simulink model "IEEE123_4subsystem"  (R2022b)
settings: Solver=ode4  StartTime=0.0  StopTime=inf  FixedStep=Ts  MaxStep=1e-4  RelTol=1e-3
PreLoadFcn:
  | Ts = 50e-6;
PostLoadFcn:
  | Ts = 50e-6;
InitFcn:
  | %%%%%%%%%%%%%%%%%%%%%%%%
  | % Simulation data for the IEEE 123 Node Test Feeder model
  | %%%%%%%%%%%%%%%%%%%%%%%
  | 
  | % miles/km
  | mi2km = 1.60934;
  | 
  | % feet to km
  | ft2km = 0.0003048;
  | 
  | % microsiemens to Farads
  | ms2F = 1/2/pi/60*1e-6;
  | 
  | %% Configuration 1 - series reactance - ohm/mile
  | 
  | R_1 = [0.4576 0.1560 0.1535;0.1560 0.4666 0.1580;0.1535 0.1580 0.4615];
  | X_1 = [1.0780 0.5017 0.3849;0.5017 1.0482 0.4236;0.3849 0.4236 1.0651];
  | 
  | % charging susceptance - microsiemens/mile
  | 
  | B_1 = [5.6765 -1.8319 -0.6982;-1.8319 5.9809 -1.1645;-0.6982 -1.1645 5.3971];
  | 
  | % convert for SPS
  | 
  | R_1 = R_1/mi2km;
  | 
  | Rs_1=(R_1(1,1)+R_1(2,2)+R_1(3,3))/3;
  | Rm_1=(R_1(1,2)+R_1(1,3)+R_1(2,3))/3;
  | R1_1=Rs_1-Rm_1;
  | R0_1=Rs_1+2*Rm_1;
  | 
  | L_1 = X_1/mi2km/2/pi/60;
  | 
  | Ls_1=(L_1(1,1)+L_1(2,2)+L_1(3,3))/3;
  | Lm_1=(L_1(1,2)+L_1(1,3)+L_1(2,3))/3;
  | L1_1=Ls_1-Lm_1;
  | L0_1=Ls_1+2*Lm_1;
  | 
  | C_1 = B_1/mi2km*ms2F;
  | 
  | Cs_1=(C_1(1,1)+C_1(2,2)+C_1(3,3))/3;
  | Cm_1=(C_1(1,2)+C_1(1,3)+C_1(2,3))/3;
  | C1_1=Cs_1-Cm_1;
  | C0_1=Cs_1+2*Cm_1;
  | 
  | 
  | %% Configuration 2 - series reactance - ohm/mile
  | 
  | R_2 = [0.4666 0.1580 0.1560;0.1580 0.4615 0.1535;0.1560 0.1535 0.4576];
  | X_2 = [1.0482 0.4236 0.5017;0.4236 1.0651 0.3849;0.5017 0.3849 1.0780];
  | 
  | % charging susceptance - microsiemens/mile
  | 
  | B_2 = [5.9809 -1.1645 -1.8319;-1.1645 5.3971 -0.6982;-1.8319 -0.6982 5.6765];
  | 
  | % convert for SPS
  | 
  | R_2 = R_2/mi2km;
  | 
  | Rs_2=(R_2(1,1)+R_2(2,2)+R_2(3,3))/3;
  | ... (+341 lines)
undefined symbols (not defined in the file): D1, Delta, find_system, I, Left, MOV_segment9, powergui, Right, type, V, X
libraries: spsGroundLib x242, spsThreePhaseVIMeasurementLib x134, spsSeriesRLCBranchLib x107, spsSeriesRLCLoadLib x83, spsPiSectionLineLib x61, spsThreePhasePISectionLineLib x60, spsVoltageMeasurementLib x52, spsDCVoltageSourceLib x36, ssn_lib x28, artemis x24, spsACCurrentSourceLib x18, spsOnDelayLib x18
(part 7 of 15)

== system IEEE123_4subsystem/SS_123p2/Regulator3 ==
  Mux : Mux  Inputs=2
  Single Phase SVR_A : Subsystem  LoadFcn=find_system(gcs,'FollowLinks', 'on', 'LookUnderMasks', 'all');  mask(Single-Phase OLTC){pNom=5e6/3, fNom=60, vNom=4160/sqrt(3), ctRatio=50, ptRatio=20, DeltaU=0.00625, TapMinMax=[-16 16], InitialTap=0, TapSelectionTime=0.2, RegulatorOn=on, Regulator=[120/120  1/120  0.2], Comp=[0.4 0.4]}
      mask prompts: pNom "Nominal Power (VA)"; fNom "Nominal Frequency (Hz)"; vNom "Nominal Voltage (Vrms)"; ctRatio "Primary CT Rating (A)"; ptRatio "PT Ratio"; DeltaU "Voltage Step Per Tap (pu)"; TapMinMax "Minimum and Maximum Tap Positions"; InitialTap "Initial Tap Position"; TapSelectionTime "Tap Selection Time (s)"; RegulatorOn "Voltage Regulator"; Regulator "Voltage Regulator [ Vref(pu) DeadBand(pu)  Delay(s)]"; Comp "Compensator Settings [R (V) X(V)]"
      mask help:
      | Models a single-phase On Load Tap Changer (OLTC). The single-phase secondary of multi-tap winding is modeled with a Variable-Ratio Transformer block.
      |
      | The transformer voltage ratio U2/U1 (in pu) is given by:
      |                 U2/U1= 1+TapPosition*DeltaU
      | Tap position 0 corresponds to nominal voltage ratio.
      |
      | When Voltage regulator is 'on',  voltage regulator asks for a tap change if:
      |                  abs(Vm-Vref)>DeadBand/2  during a time  t > Delay.
      |
      | where 'Vm' is voltage measured at regulating point and Vref is reference voltage.
      | With line drop compensation, Vm=Vsec-Isec(R+jX)
      mask init:
      | RegulatorVref=Regulator(1);
      | RegulatorDeadBand=Regulator(2);
      | RegulatorDelay=Regulator(3);
      | Rc=Comp(1);
      | Xc=Comp(2);
      mask TypeOptions RegulatorOn: off | on
      mask Callback RegulatorOn:
      | tempMaskVis=get_param(gcb,'MaskVisibilities');
      | if strcmp(get_param(gcb,'RegulatorOn'),'on')
      | 	tempMaskVis{11}='on';
      | 	set_param(gcb,'MaskVisibilities',tempMaskVis);
      | else
      | 	tempMaskVis{11}='off';
      | 	set_param(gcb,'MaskVisibilities',tempMaskVis);
      | end
      | if strcmp(get_param(gcb,'RegulatorOn'),'on')
      | 	tempMaskVis{12}='on';
      | 	set_param(gcb,'MaskVisibilities',tempMaskVis);
      | else
      | 	tempMaskVis{12}='off';
      | 	set_param(gcb,'MaskVisibilities',tempMaskVis);
      | end
      mask DialogControl Container8 Prompt: Setup
      mask DialogControl Container13 Prompt: Regulator Parameters
      mask Display:
      | color('green');
      | r=50;x=40;y=80;
      | th = 0:pi/100:2*pi;
      | f = r * exp(j*th) + x+j*y;
      | plot(real(f), imag(f));
      | color('blue');
      | plot([-10 90],[30,130])
      | plot([75 90],[125,130])
      | plot([85 90],[115,130])
      | color('black')
      | port_label('Lconn',1,'S');port_label('Rconn',1,'L');
      | text(58,115,'Tap');
      | text(43,70,'Vsec');
      | text(48,95,'Isec');
  Single Phase SVR_C : Subsystem  LoadFcn=find_system(gcs,'FollowLinks', 'on', 'LookUnderMasks', 'all');  mask(Single-Phase OLTC){pNom=5e6/3, fNom=60, vNom=4160/sqrt(3), ctRatio=50, ptRatio=20, DeltaU=0.00625, TapMinMax=[-16 16], InitialTap=-1, TapSelectionTime=0.2, RegulatorOn=on, Regulator=[120/120  1/120  0.2], Comp=[0.4 0.4]}
      mask prompts: pNom "Nominal Power (VA)"; fNom "Nominal Frequency (Hz)"; vNom "Nominal Voltage (Vrms)"; ctRatio "Primary CT Rating (A)"; ptRatio "PT Ratio"; DeltaU "Voltage Step Per Tap (pu)"; TapMinMax "Minimum and Maximum Tap Positions"; InitialTap "Initial Tap Position"; TapSelectionTime "Tap Selection Time (s)"; RegulatorOn "Voltage Regulator"; Regulator "Voltage Regulator [ Vref(pu) DeadBand(pu)  Delay(s)]"; Comp "Compensator Settings [R (V) X(V)]"
      mask help:
      | Models a single-phase On Load Tap Changer (OLTC). The single-phase secondary of multi-tap winding is modeled with a Variable-Ratio Transformer block.
      |
      | The transformer voltage ratio U2/U1 (in pu) is given by:
      |                 U2/U1= 1+TapPosition*DeltaU
      | Tap position 0 corresponds to nominal voltage ratio.
      |
      | When Voltage regulator is 'on',  voltage regulator asks for a tap change if:
      |                  abs(Vm-Vref)>DeadBand/2  during a time  t > Delay.
      |
      | where 'Vm' is voltage measured at regulating point and Vref is reference voltage.
      | With line drop compensation, Vm=Vsec-Isec(R+jX)
      mask init:
      | RegulatorVref=Regulator(1);
      | RegulatorDeadBand=Regulator(2);
      | RegulatorDelay=Regulator(3);
      | Rc=Comp(1);
      | Xc=Comp(2);
      mask TypeOptions RegulatorOn: off | on
      mask Callback RegulatorOn:
      | tempMaskVis=get_param(gcb,'MaskVisibilities');
      | if strcmp(get_param(gcb,'RegulatorOn'),'on')
      | 	tempMaskVis{11}='on';
      | 	set_param(gcb,'MaskVisibilities',tempMaskVis);
      | else
      | 	tempMaskVis{11}='off';
      | 	set_param(gcb,'MaskVisibilities',tempMaskVis);
      | end
      | if strcmp(get_param(gcb,'RegulatorOn'),'on')
      | 	tempMaskVis{12}='on';
      | 	set_param(gcb,'MaskVisibilities',tempMaskVis);
      | else
      | 	tempMaskVis{12}='off';
      | 	set_param(gcb,'MaskVisibilities',tempMaskVis);
      | end
      mask DialogControl Container8 Prompt: Setup
      mask DialogControl Container13 Prompt: Regulator Parameters
      mask Display:
      | color('green');
      | r=50;x=40;y=80;
      | th = 0:pi/100:2*pi;
      | f = r * exp(j*th) + x+j*y;
      | plot(real(f), imag(f));
      | color('blue');
      | plot([-10 90],[30,130])
      | plot([75 90],[125,130])
      | plot([85 90],[115,130])
      | color('black')
      | port_label('Lconn',1,'S');port_label('Rconn',1,'L');
      | text(58,115,'Tap');
      | text(43,70,'Vsec');
      | text(48,95,'Isec');
  A : PMIOPort  Side=Left
  a : PMIOPort  Port=2  Side=Right
  C : PMIOPort  Port=3  Side=Left
  c : PMIOPort  Port=4  Side=Right
  Taps : Outport
  wires:
  Single Phase SVR_A/1(Tap) -> Mux/1
  Single Phase SVR_C/1(Tap) -> Mux/2
  Mux/1 -> Taps/1
  connections:
  Single Phase SVR_A/LConn1 -- A/RConn1
  Single Phase SVR_C/LConn1 -- C/RConn1
  Single Phase SVR_A/RConn1 -- a/RConn1
  Single Phase SVR_C/RConn1 -- c/RConn1

== system IEEE123_4subsystem/SS_123p3/68 ==
  2 : spsThreePhaseVIMeasurementLib/Three-Phase V-I Measurement  VoltageMeasurement=phase-to-ground  SetLabelV=on  LabelV=V68  Vpu=off  VpuLL=off  CurrentMeasurement=no  SetLabelI=on  LabelI=I800  Ipu=off  Pbase=100e6  Vbase=24900  OutputType=Complex  PhasorSimulation=off  PSBequivalent=0
  Ground82 : spsGroundLib/Ground  LConnTagsString=a
  Ground83 : spsGroundLib/Ground  LConnTagsString=a
  a : PMIOPort  Side=Right
  A : PMIOPort  Port=2  Side=Left
  connections:
  A/RConn1 -- 2/LConn1
  a/RConn1 -- 2/RConn1
  Ground83/LConn1 -- 2/LConn2 -- 2/LConn3
  Ground82/LConn1 -- 2/RConn2 -- 2/RConn3

== system IEEE123_4subsystem/SS_123p3/69 ==
  2 : spsThreePhaseVIMeasurementLib/Three-Phase V-I Measurement  VoltageMeasurement=phase-to-ground  SetLabelV=on  LabelV=V69  Vpu=off  VpuLL=off  CurrentMeasurement=no  SetLabelI=on  LabelI=I800  Ipu=off  Pbase=100e6  Vbase=24900  OutputType=Complex  PhasorSimulation=off  PSBequivalent=0
  Ground82 : spsGroundLib/Ground  LConnTagsString=a
  Ground83 : spsGroundLib/Ground  LConnTagsString=a
  a : PMIOPort  Side=Right
  A : PMIOPort  Port=2  Side=Left
  connections:
  2/RConn3 -- 2/RConn2 -- Ground82/LConn1
  2/LConn3 -- 2/LConn2 -- Ground83/LConn1
  a/RConn1 -- 2/RConn1
  A/RConn1 -- 2/LConn1

== system IEEE123_4subsystem/SS_123p3/70 ==
  2 : spsThreePhaseVIMeasurementLib/Three-Phase V-I Measurement  VoltageMeasurement=phase-to-ground  SetLabelV=on  LabelV=V70  Vpu=off  VpuLL=off  CurrentMeasurement=no  SetLabelI=on  LabelI=I800  Ipu=off  Pbase=100e6  Vbase=24900  OutputType=Complex  PhasorSimulation=off  PSBequivalent=0
  Ground82 : spsGroundLib/Ground  LConnTagsString=a
  Ground83 : spsGroundLib/Ground  LConnTagsString=a
  a : PMIOPort  Side=Right
  A : PMIOPort  Port=2  Side=Left
  connections:
  A/RConn1 -- 2/LConn1
  a/RConn1 -- 2/RConn1
  Ground83/LConn1 -- 2/LConn2 -- 2/LConn3
  Ground82/LConn1 -- 2/RConn2 -- 2/RConn3

== system IEEE123_4subsystem/SS_123p3/71 ==
  2 : spsThreePhaseVIMeasurementLib/Three-Phase V-I Measurement  VoltageMeasurement=phase-to-ground  SetLabelV=on  LabelV=V71  Vpu=off  VpuLL=off  CurrentMeasurement=no  SetLabelI=on  LabelI=I800  Ipu=off  Pbase=100e6  Vbase=24900  OutputType=Complex  PhasorSimulation=off  PSBequivalent=0
  Ground82 : spsGroundLib/Ground  LConnTagsString=a
  Ground83 : spsGroundLib/Ground  LConnTagsString=a
  a : PMIOPort  Side=Right
  A : PMIOPort  Port=2  Side=Left
  connections:
  2/RConn3 -- 2/RConn2 -- Ground82/LConn1
  2/LConn3 -- 2/LConn2 -- Ground83/LConn1
  a/RConn1 -- 2/RConn1
  A/RConn1 -- 2/LConn1

== system IEEE123_4subsystem/SS_123p3/73 ==
  2 : spsThreePhaseVIMeasurementLib/Three-Phase V-I Measurement  VoltageMeasurement=phase-to-ground  SetLabelV=on  LabelV=V73  Vpu=off  VpuLL=off  CurrentMeasurement=no  SetLabelI=on  LabelI=I800  Ipu=off  Pbase=100e6  Vbase=24900  OutputType=Complex  PhasorSimulation=off  PSBequivalent=0
  Ground82 : spsGroundLib/Ground  LConnTagsString=a
  Ground83 : spsGroundLib/Ground  LConnTagsString=a
  c : PMIOPort  Side=Right
  C : PMIOPort  Port=2  Side=Left
  connections:
  2/LConn1 -- 2/LConn2 -- Ground83/LConn1
  2/RConn1 -- 2/RConn2 -- Ground82/LConn1
  c/RConn1 -- 2/RConn3
  C/RConn1 -- 2/LConn3

== system IEEE123_4subsystem/SS_123p3/74 ==
  2 : spsThreePhaseVIMeasurementLib/Three-Phase V-I Measurement  VoltageMeasurement=phase-to-ground  SetLabelV=on  LabelV=V74  Vpu=off  VpuLL=off  CurrentMeasurement=no  SetLabelI=on  LabelI=I800  Ipu=off  Pbase=100e6  Vbase=24900  OutputType=Complex  PhasorSimulation=off  PSBequivalent=0
  Ground82 : spsGroundLib/Ground  LConnTagsString=a
  Ground83 : spsGroundLib/Ground  LConnTagsString=a
  c : PMIOPort  Side=Right
  C : PMIOPort  Port=2  Side=Left
  connections:
  C/RConn1 -- 2/LConn3
  c/RConn1 -- 2/RConn3
  Ground82/LConn1 -- 2/RConn2 -- 2/RConn1
  Ground83/LConn1 -- 2/LConn2 -- 2/LConn1

== system IEEE123_4subsystem/SS_123p3/75 ==
  2 : spsThreePhaseVIMeasurementLib/Three-Phase V-I Measurement  VoltageMeasurement=phase-to-ground  SetLabelV=on  LabelV=V75  Vpu=off  VpuLL=off  CurrentMeasurement=no  SetLabelI=on  LabelI=I800  Ipu=off  Pbase=100e6  Vbase=24900  OutputType=Complex  PhasorSimulation=off  PSBequivalent=0
  Ground82 : spsGroundLib/Ground  LConnTagsString=a
  Ground83 : spsGroundLib/Ground  LConnTagsString=a
  c : PMIOPort  Side=Right
  C : PMIOPort  Port=2  Side=Left
  connections:
  2/LConn1 -- 2/LConn2 -- Ground83/LConn1
  2/RConn1 -- 2/RConn2 -- Ground82/LConn1
  c/RConn1 -- 2/RConn3
  C/RConn1 -- 2/LConn3

== system IEEE123_4subsystem/SS_123p3/84 ==
  2 : spsThreePhaseVIMeasurementLib/Three-Phase V-I Measurement  VoltageMeasurement=phase-to-ground  SetLabelV=on  LabelV=V84  Vpu=off  VpuLL=off  CurrentMeasurement=no  SetLabelI=on  LabelI=I800  Ipu=off  Pbase=100e6  Vbase=24900  OutputType=Complex  PhasorSimulation=off  PSBequivalent=0
  Ground82 : spsGroundLib/Ground  LConnTagsString=a
  Ground83 : spsGroundLib/Ground  LConnTagsString=a
  c : PMIOPort  Side=Right
  C : PMIOPort  Port=2  Side=Left
  connections:
  C/RConn1 -- 2/LConn3
  c/RConn1 -- 2/RConn3
  Ground82/LConn1 -- 2/RConn2 -- 2/RConn1
  Ground83/LConn1 -- 2/LConn2 -- 2/LConn1

== system IEEE123_4subsystem/SS_123p3/85 ==
  2 : spsThreePhaseVIMeasurementLib/Three-Phase V-I Measurement  VoltageMeasurement=phase-to-ground  SetLabelV=on  LabelV=V85  Vpu=off  VpuLL=off  CurrentMeasurement=no  SetLabelI=on  LabelI=I800  Ipu=off  Pbase=100e6  Vbase=24900  OutputType=Complex  PhasorSimulation=off  PSBequivalent=0
  Ground82 : spsGroundLib/Ground  LConnTagsString=a
  Ground83 : spsGroundLib/Ground  LConnTagsString=a
  c : PMIOPort  Side=Right
  C : PMIOPort  Port=2  Side=Left
  connections:
  2/LConn1 -- 2/LConn2 -- Ground83/LConn1
  2/RConn1 -- 2/RConn2 -- Ground82/LConn1
  c/RConn1 -- 2/RConn3
  C/RConn1 -- 2/LConn3

== system IEEE123_4subsystem/SS_123p3/88 ==
  2 : spsThreePhaseVIMeasurementLib/Three-Phase V-I Measurement  VoltageMeasurement=phase-to-ground  SetLabelV=on  LabelV=V88  Vpu=off  VpuLL=off  CurrentMeasurement=no  SetLabelI=on  LabelI=I800  Ipu=off  Pbase=100e6  Vbase=24900  OutputType=Complex  PhasorSimulation=off  PSBequivalent=0
  Ground82 : spsGroundLib/Ground  LConnTagsString=a
  Ground83 : spsGroundLib/Ground  LConnTagsString=a
  a : PMIOPort  Side=Right
  A : PMIOPort  Port=2  Side=Left
  connections:
  A/RConn1 -- 2/LConn1
  a/RConn1 -- 2/RConn1
  2/LConn2 -- 2/LConn3 -- Ground83/LConn1
  2/RConn2 -- 2/RConn3 -- Ground82/LConn1

== system IEEE123_4subsystem/SS_123p3/90 ==
  2 : spsThreePhaseVIMeasurementLib/Three-Phase V-I Measurement  VoltageMeasurement=phase-to-ground  SetLabelV=on  LabelV=V90  Vpu=off  VpuLL=off  CurrentMeasurement=no  SetLabelI=on  LabelI=I800  Ipu=off  Pbase=100e6  Vbase=24900  OutputType=Complex  PhasorSimulation=off  PSBequivalent=0
  Ground82 : spsGroundLib/Ground  LConnTagsString=a
  Ground83 : spsGroundLib/Ground  LConnTagsString=a
  b : PMIOPort  Side=Right
  B : PMIOPort  Port=2  Side=Left
  connections:
  Ground82/LConn1 -- 2/RConn3 -- 2/RConn1
  Ground83/LConn1 -- 2/LConn3 -- 2/LConn1
  2/RConn2 -- b/RConn1
  2/LConn2 -- B/RConn1

== system IEEE123_4subsystem/SS_123p3/92 ==
  2 : spsThreePhaseVIMeasurementLib/Three-Phase V-I Measurement  VoltageMeasurement=phase-to-ground  SetLabelV=on  LabelV=V92  Vpu=off  VpuLL=off  CurrentMeasurement=no  SetLabelI=on  LabelI=I800  Ipu=off  Pbase=100e6  Vbase=24900  OutputType=Complex  PhasorSimulation=off  PSBequivalent=0
  Ground82 : spsGroundLib/Ground  LConnTagsString=a
  Ground83 : spsGroundLib/Ground  LConnTagsString=a
  c : PMIOPort  Side=Right
  C : PMIOPort  Port=2  Side=Left
  connections:
  C/RConn1 -- 2/LConn3
  c/RConn1 -- 2/RConn3
  2/RConn2 -- 2/RConn1 -- Ground82/LConn1
  2/LConn2 -- 2/LConn1 -- Ground83/LConn1

== system IEEE123_4subsystem/SS_123p3/94 ==
  2 : spsThreePhaseVIMeasurementLib/Three-Phase V-I Measurement  VoltageMeasurement=phase-to-ground  SetLabelV=on  LabelV=V94  Vpu=off  VpuLL=off  CurrentMeasurement=no  SetLabelI=on  LabelI=I800  Ipu=off  Pbase=100e6  Vbase=24900  OutputType=Complex  PhasorSimulation=off  PSBequivalent=0
  Ground82 : spsGroundLib/Ground  LConnTagsString=a
  Ground83 : spsGroundLib/Ground  LConnTagsString=a
  a : PMIOPort  Side=Right
  A : PMIOPort  Port=2  Side=Left
  connections:
  Ground82/LConn1 -- 2/RConn3 -- 2/RConn2
  Ground83/LConn1 -- 2/LConn3 -- 2/LConn2
  a/RConn1 -- 2/RConn1
  A/RConn1 -- 2/LConn1

== system IEEE123_4subsystem/SS_123p3/96 ==
  2 : spsThreePhaseVIMeasurementLib/Three-Phase V-I Measurement  VoltageMeasurement=phase-to-ground  SetLabelV=on  LabelV=V96  Vpu=off  VpuLL=off  CurrentMeasurement=no  SetLabelI=on  LabelI=I800  Ipu=off  Pbase=100e6  Vbase=24900  OutputType=Complex  PhasorSimulation=off  PSBequivalent=0
  Ground82 : spsGroundLib/Ground  LConnTagsString=a
  Ground83 : spsGroundLib/Ground  LConnTagsString=a
  b : PMIOPort  Side=Right
  B : PMIOPort  Port=2  Side=Left
  connections:
  2/LConn2 -- B/RConn1
  2/RConn2 -- b/RConn1
  2/LConn1 -- 2/LConn3 -- Ground83/LConn1
  2/RConn1 -- 2/RConn3 -- Ground82/LConn1

== system IEEE123_4subsystem/powergui/EquivalentModel1 ==
  Sources : Subsystem
  State-Space : S-Function  FunctionName=ssn_sfun_v1  Parameters=1,0  SFunctionDeploymentMode=off  EnableBusSupport=off  SFcnStateName=MOV_segment9,MOV_segment9,MOV_segment9,MOV_segment9,MOV_segment9,MOV_segment9,MOV_segment9,MOV_segment9,MOV_segment9,MOV_segment9
      settings: SFcnIsStateOwnerBlock=on
  Yout : Subsystem
  wires:
  State-Space/1 -> Yout/1(v,i)
  Sources/1(u) -> State-Space/1

== system IEEE123_4subsystem/powergui/EquivalentModel10 ==
  Gates : Subsystem
  Sources : Subsystem
  State-Space : Subsystem
  Status : Subsystem
  Yout : Subsystem
  wires:
  Gates/1(gates) -> State-Space/2(In2)
  Sources/1(u) -> State-Space/1(In1)
  State-Space/2(Out2) -> Status/1(status)
  State-Space/1(Out1) -> Yout/1(v,i)

== system IEEE123_4subsystem/powergui/EquivalentModel11 ==
  Gates : Subsystem
  Sources : Subsystem
  State-Space : Subsystem
  Status : Subsystem
  Yout : Subsystem
  wires:
  Gates/1(gates) -> State-Space/2(In2)
  Sources/1(u) -> State-Space/1(In1)
  State-Space/2(Out2) -> Status/1(status)
  State-Space/1(Out1) -> Yout/1(v,i)

== system IEEE123_4subsystem/powergui/EquivalentModel2 ==
  Sources : Subsystem
  State-Space : S-Function  FunctionName=ssn_sfun_v1  Parameters=2,0  SFunctionDeploymentMode=off  EnableBusSupport=off  SFcnStateName=MOV_segment9,MOV_segment9,MOV_segment9,MOV_segment9,MOV_segment9,MOV_segment9,MOV_segment9,MOV_segment9,MOV_segment9,MOV_segment9
      settings: SFcnIsStateOwnerBlock=on
  Yout : Subsystem
  wires:
  State-Space/1 -> Yout/1(v,i)
  Sources/1(u) -> State-Space/1

== system IEEE123_4subsystem/powergui/EquivalentModel3 ==
  Sources : Subsystem
  State-Space : S-Function  FunctionName=ssn_sfun_v1  Parameters=3,0  SFunctionDeploymentMode=off  EnableBusSupport=off  SFcnStateName=MOV_segment9,MOV_segment9,MOV_segment9,MOV_segment9,MOV_segment9,MOV_segment9,MOV_segment9,MOV_segment9,MOV_segment9,MOV_segment9
      settings: SFcnIsStateOwnerBlock=on
  Yout : Subsystem
  wires:
  State-Space/1 -> Yout/1(v,i)
  Sources/1(u) -> State-Space/1

== system IEEE123_4subsystem/powergui/EquivalentModel4 ==
  Sources : Subsystem
  State-Space : S-Function  FunctionName=ssn_sfun_v1  Parameters=4,0  SFunctionDeploymentMode=off  EnableBusSupport=off  SFcnStateName=MOV_segment9,MOV_segment9,MOV_segment9,MOV_segment9,MOV_segment9,MOV_segment9,MOV_segment9,MOV_segment9,MOV_segment9,MOV_segment9
      settings: SFcnIsStateOwnerBlock=on
  Yout : Subsystem
  wires:
  State-Space/1 -> Yout/1(v,i)
  Sources/1(u) -> State-Space/1

== system IEEE123_4subsystem/powergui/EquivalentModel5 ==
  Sources : Subsystem
  State-Space : S-Function  FunctionName=ssn_sfun_v1  Parameters=5,0  SFunctionDeploymentMode=off  EnableBusSupport=off  SFcnStateName=MOV_segment9,MOV_segment9,MOV_segment9,MOV_segment9,MOV_segment9,MOV_segment9,MOV_segment9,MOV_segment9,MOV_segment9,MOV_segment9
      settings: SFcnIsStateOwnerBlock=on
  Yout : Subsystem
  wires:
  State-Space/1 -> Yout/1(v,i)
  Sources/1(u) -> State-Space/1

== system IEEE123_4subsystem/powergui/EquivalentModel6 ==
  Sources : Subsystem
  State-Space : S-Function  FunctionName=ssn_sfun_v1  Parameters=6,0  SFunctionDeploymentMode=off  EnableBusSupport=off  SFcnStateName=MOV_segment9,MOV_segment9,MOV_segment9,MOV_segment9,MOV_segment9,MOV_segment9,MOV_segment9,MOV_segment9,MOV_segment9,MOV_segment9
      settings: SFcnIsStateOwnerBlock=on
  Yout : Subsystem
  wires:
  State-Space/1 -> Yout/1(v,i)
  Sources/1(u) -> State-Space/1

== system IEEE123_4subsystem/powergui/EquivalentModel7 ==
  Sources : Subsystem
  State-Space : S-Function  FunctionName=ssn_sfun_v1  Parameters=7,0  SFunctionDeploymentMode=off  EnableBusSupport=off  SFcnStateName=MOV_segment9,MOV_segment9,MOV_segment9,MOV_segment9,MOV_segment9,MOV_segment9,MOV_segment9,MOV_segment9,MOV_segment9,MOV_segment9
      settings: SFcnIsStateOwnerBlock=on
  Yout : Subsystem
  wires:
  State-Space/1 -> Yout/1(v,i)
  Sources/1(u) -> State-Space/1

== system IEEE123_4subsystem/powergui/EquivalentModel8 ==
  Sources : Subsystem
  State-Space : S-Function  FunctionName=ssn_sfun_v1  Parameters=8,0  SFunctionDeploymentMode=off  EnableBusSupport=off  SFcnStateName=MOV_segment9,MOV_segment9,MOV_segment9,MOV_segment9,MOV_segment9,MOV_segment9,MOV_segment9,MOV_segment9,MOV_segment9,MOV_segment9
      settings: SFcnIsStateOwnerBlock=on
  Yout : Subsystem
  wires:
  State-Space/1 -> Yout/1(v,i)
  Sources/1(u) -> State-Space/1

== system IEEE123_4subsystem/powergui/EquivalentModel9 ==
  Gates : Subsystem
  Sources : Subsystem
  State-Space : Subsystem
  Status : Subsystem
  Yout : Subsystem
  wires:
  Gates/1(gates) -> State-Space/2(In2)
  Sources/1(u) -> State-Space/1(In1)
  State-Space/2(Out2) -> Status/1(status)
  State-Space/1(Out1) -> Yout/1(v,i)

== system IEEE123_4subsystem/SM_123p/Regulator 1 Three Phase Ganged SVR/Ganged Line Drop Compensator ==
  note: Vm=Vsec-Isec(Rc+jXc)
  Isec : Inport
  Vsec : Inport  Port=2
  "        " : spsLinearTransformerLib/Linear Transformer  UNITS=SI  NominalPower=[pNom fNom]  winding1=[vNom/ptRatio 1e-7 1e-8]  winding2=[vNom/ptRatio 1e-7 1e-8]  ThreeWindings=off  winding3=[3.15e+005 0.7938 0.084225]  RmLm=[1e5 1e5]  Measurements=None  DataType=on
  "CTS  " : spsControlledCurrentSourceLib/Controlled Current Source  Initialize=on  Source_Type=AC  Amplitude=0  Phase=0  Frequency=0  Measurements=None
  "PTS  " : spsControlledVoltageSourceLib/Controlled Voltage Source  Initialize=on  Source_Type=AC  Amplitude=0  Phase=0  Frequency=0  Measurements=None
  RMS : spsRMSLib/RMS  TrueRMS=on  Freq=60  RMSInit=120  Ts=0
  Raux : spsSeriesRLCBranchLib/Series RLC Branch  LConnTagsString=__new0  RConnTagsString=__new0  BranchType=R  Resistance=1e3  Inductance=1.6 / (120*pi)  SetiL0=off  InitialCurrent=0  Capacitance=1e-6  Setx0=off  InitialVoltage=0  Measurements=None
  Rc+jXc : spsSeriesRLCBranchLib/Series RLC Branch  LConnTagsString=__new0  RConnTagsString=__new0  BranchType=RL  Resistance=Rc  Inductance=Xc / (2*pi*fNom)  SetiL0=off  InitialCurrent=0  Capacitance=1e-6  Setx0=off  InitialVoltage=0  Measurements=None
  VRelay : spsVoltageMeasurementLib/Voltage Measurement  PhasorSimulation=off  OutputType=Complex  PSBequivalent=0
  Vm : Outport
  wires:
  Vsec/1 -> "PTS  "/1
  Isec/1 -> "CTS  "/1
  VRelay/1 -> RMS/1
  RMS/1 -> Vm/1
  connections:
  VRelay/LConn2 -- "PTS  "/LConn1
  "        "/LConn2 -- "CTS  "/LConn1 -- Raux/RConn1 -- Rc+jXc/RConn1
  "CTS  "/RConn1 -- "        "/LConn1 -- Rc+jXc/LConn1 -- Raux/LConn1
  "        "/RConn2 -- VRelay/LConn1
  "PTS  "/RConn1 -- "        "/RConn1

== system IEEE123_4subsystem/SM_123p/Regulator 1 Three Phase Ganged SVR/Single Phase SVR_A ==
  Vm : Inport
  Transformer with Taps : Subsystem
  Voltage Regulator Control : Subsystem
  S : PMIOPort  Tag=PMCPort  Side=Left
  L : PMIOPort  Tag=PMCPort  Port=2  Side=Right
  Tap : Outport  VectorParamsAs1DForOutWhenUnconnected=off
  Isec : Outport  Port=2  VectorParamsAs1DForOutWhenUnconnected=off
  Vsec : Outport  Port=3  VectorParamsAs1DForOutWhenUnconnected=off
  wires:
  Transformer with Taps/2(Vsec) -> Vsec/1
  Transformer with Taps/1(Isec) -> Isec/1
  Voltage Regulator Control/1(N) -> Transformer with Taps/1(N)
  Voltage Regulator Control/2(Tap) -> Tap/1
  Vm/1 -> Voltage Regulator Control/1(Vm)
  connections:
  S/RConn1 -- Transformer with Taps/LConn1
  Transformer with Taps/RConn1 -- L/RConn1

== system IEEE123_4subsystem/SM_123p/Regulator 1 Three Phase Ganged SVR/Single Phase SVR_B ==
  Vm : Inport
  Transformer with Taps : Subsystem
  Voltage Regulator Control : Subsystem
  S : PMIOPort  Tag=PMCPort  Side=Left
  L : PMIOPort  Tag=PMCPort  Port=2  Side=Right
  Tap : Outport  VectorParamsAs1DForOutWhenUnconnected=off
  Isec : Outport  Port=2  VectorParamsAs1DForOutWhenUnconnected=off
  Vsec : Outport  Port=3  VectorParamsAs1DForOutWhenUnconnected=off
  wires:
  Vm/1 -> Voltage Regulator Control/1(Vm)
  Voltage Regulator Control/2(Tap) -> Tap/1
  Voltage Regulator Control/1(N) -> Transformer with Taps/1(N)
  Transformer with Taps/1(Isec) -> Isec/1
  Transformer with Taps/2(Vsec) -> Vsec/1
  connections:
  Transformer with Taps/RConn1 -- L/RConn1
  Transformer with Taps/LConn1 -- S/RConn1

== system IEEE123_4subsystem/SM_123p/Regulator 1 Three Phase Ganged SVR/Single Phase SVR_C ==
  Vm : Inport
  Transformer with Taps : Subsystem
  Voltage Regulator Control : Subsystem
  S : PMIOPort  Tag=PMCPort  Side=Left
  L : PMIOPort  Tag=PMCPort  Port=2  Side=Right
  Tap : Outport  VectorParamsAs1DForOutWhenUnconnected=off
  Isec : Outport  Port=2  VectorParamsAs1DForOutWhenUnconnected=off
  Vsec : Outport  Port=3  VectorParamsAs1DForOutWhenUnconnected=off
  wires:
  Transformer with Taps/2(Vsec) -> Vsec/1
  Transformer with Taps/1(Isec) -> Isec/1
  Voltage Regulator Control/1(N) -> Transformer with Taps/1(N)
  Voltage Regulator Control/2(Tap) -> Tap/1
  Vm/1 -> Voltage Regulator Control/1(Vm)
  connections:
  Transformer with Taps/LConn1 -- S/RConn1
  Transformer with Taps/RConn1 -- L/RConn1

== system IEEE123_4subsystem/SM_123p/Regulator 2/Single Phase SVR_A ==
  Line Drop Compensator : Subsystem
  Transformer with Taps : Subsystem
  Voltage Regulator Control : Subsystem
  S : PMIOPort  Tag=PMCPort  Side=Left
  L : PMIOPort  Tag=PMCPort  Port=2  Side=Right
  Tap : Outport  VectorParamsAs1DForOutWhenUnconnected=off
  tag scope: Vr2a=global
  wires:
  Line Drop Compensator/1(Vm) -> Voltage Regulator Control/1(Vm), [Vr2a]
  Voltage Regulator Control/2(Tap) -> Tap/1
  Voltage Regulator Control/1(N) -> Transformer with Taps/1(N)
  Transformer with Taps/1(Isec) -> Line Drop Compensator/1(Isec)
  Transformer with Taps/2(Vsec) -> Line Drop Compensator/2(Vsec)
  connections:
  Transformer with Taps/RConn1 -- L/RConn1
  Transformer with Taps/LConn1 -- S/RConn1

== system IEEE123_4subsystem/SS_123p1/Regulator 4/Single Phase SVR_A ==
  Line Drop Compensator : Subsystem
  Transformer with Taps : Subsystem
  Voltage Regulator Control : Subsystem
  S : PMIOPort  Tag=PMCPort  Side=Left
  L : PMIOPort  Tag=PMCPort  Port=2  Side=Right
  Tap : Outport  VectorParamsAs1DForOutWhenUnconnected=off
  tag scope: Vr4a=global
  wires:
  Line Drop Compensator/1(Vm) -> Voltage Regulator Control/1(Vm), [Vr4a]
  Voltage Regulator Control/2(Tap) -> Tap/1
  Voltage Regulator Control/1(N) -> Transformer with Taps/1(N)
  Transformer with Taps/1(Isec) -> Line Drop Compensator/1(Isec)
  Transformer with Taps/2(Vsec) -> Line Drop Compensator/2(Vsec)
  connections:
  Transformer with Taps/RConn1 -- L/RConn1
  Transformer with Taps/LConn1 -- S/RConn1

== system IEEE123_4subsystem/SS_123p1/Regulator 4/Single Phase SVR_B ==
  Line Drop Compensator : Subsystem
  Transformer with Taps : Subsystem
  Voltage Regulator Control : Subsystem
  S : PMIOPort  Tag=PMCPort  Side=Left
  L : PMIOPort  Tag=PMCPort  Port=2  Side=Right
  Tap : Outport  VectorParamsAs1DForOutWhenUnconnected=off
  tag scope: Vr4b=global
  wires:
  Transformer with Taps/2(Vsec) -> Line Drop Compensator/2(Vsec)
  Transformer with Taps/1(Isec) -> Line Drop Compensator/1(Isec)
  Voltage Regulator Control/1(N) -> Transformer with Taps/1(N)
  Voltage Regulator Control/2(Tap) -> Tap/1
  Line Drop Compensator/1(Vm) -> Voltage Regulator Control/1(Vm), [Vr4b]
  connections:
  Transformer with Taps/LConn1 -- S/RConn1
  Transformer with Taps/RConn1 -- L/RConn1

== system IEEE123_4subsystem/SS_123p1/Regulator 4/Single Phase SVR_C ==
  Line Drop Compensator : Subsystem
  Transformer with Taps : Subsystem
  Voltage Regulator Control : Subsystem
  S : PMIOPort  Tag=PMCPort  Side=Left
  L : PMIOPort  Tag=PMCPort  Port=2  Side=Right
  Tap : Outport  VectorParamsAs1DForOutWhenUnconnected=off
  tag scope: Vr4c=global
  wires:
  Line Drop Compensator/1(Vm) -> Voltage Regulator Control/1(Vm), [Vr4c]
  Voltage Regulator Control/2(Tap) -> Tap/1
  Voltage Regulator Control/1(N) -> Transformer with Taps/1(N)
  Transformer with Taps/1(Isec) -> Line Drop Compensator/1(Isec)
  Transformer with Taps/2(Vsec) -> Line Drop Compensator/2(Vsec)
  connections:
  Transformer with Taps/RConn1 -- L/RConn1
  Transformer with Taps/LConn1 -- S/RConn1

== system IEEE123_4subsystem/SS_123p2/Regulator3/Single Phase SVR_A ==
  Line Drop Compensator : Subsystem
  Transformer with Taps : Subsystem
  Voltage Regulator Control : Subsystem
  S : PMIOPort  Tag=PMCPort  Side=Left
  L : PMIOPort  Tag=PMCPort  Port=2  Side=Right
  Tap : Outport  VectorParamsAs1DForOutWhenUnconnected=off
  tag scope: Vr3a=global
  wires:
  Line Drop Compensator/1(Vm) -> Voltage Regulator Control/1(Vm), [Vr3a]
  Voltage Regulator Control/2(Tap) -> Tap/1
  Voltage Regulator Control/1(N) -> Transformer with Taps/1(N)
  Transformer with Taps/1(Isec) -> Line Drop Compensator/1(Isec)
  Transformer with Taps/2(Vsec) -> Line Drop Compensator/2(Vsec)
  connections:
  Transformer with Taps/RConn1 -- L/RConn1
  Transformer with Taps/LConn1 -- S/RConn1

== system IEEE123_4subsystem/SS_123p2/Regulator3/Single Phase SVR_C ==
  Line Drop Compensator : Subsystem
  Transformer with Taps : Subsystem
  Voltage Regulator Control : Subsystem
  S : PMIOPort  Tag=PMCPort  Side=Left
  L : PMIOPort  Tag=PMCPort  Port=2  Side=Right
  Tap : Outport  VectorParamsAs1DForOutWhenUnconnected=off
  tag scope: Vr3c=global
  wires:
  Transformer with Taps/2(Vsec) -> Line Drop Compensator/2(Vsec)
  Transformer with Taps/1(Isec) -> Line Drop Compensator/1(Isec)
  Voltage Regulator Control/1(N) -> Transformer with Taps/1(N)
  Voltage Regulator Control/2(Tap) -> Tap/1
  Line Drop Compensator/1(Vm) -> Voltage Regulator Control/1(Vm), [Vr3c]
  connections:
  Transformer with Taps/LConn1 -- S/RConn1
  Transformer with Taps/RConn1 -- L/RConn1

== system IEEE123_4subsystem/powergui/EquivalentModel1/Sources ==
  Mux : Mux  Inputs=[1 1]
  u : Outport  VectorParamsAs1DForOutWhenUnconnected=off
  wires:
  Mux/1 -> u/1
  [T101_8664_15937078016277] -> Mux/1
  [T101_8651_15842475818836] -> Mux/2

== system IEEE123_4subsystem/powergui/EquivalentModel1/Yout ==
  v,i : Inport
  Demux : Demux  Outputs=1
  tag scope: T104_9196_19269757098139=global
  wires:
  v,i/1 -> Demux/1
  Demux/1 -> [T104_9196_19269757098139]

== system IEEE123_4subsystem/powergui/EquivalentModel10/Gates ==
  Mux : Mux  Inputs=[1 1 1 1 1 1]
  gates : Outport  VectorParamsAs1DForOutWhenUnconnected=off
  wires:
  Mux/1 -> gates/1
  [T48_3792_3444493035527] -> Mux/1
  [T48_3793_3447166059747] -> Mux/2
  [T48_3794_3449967890634] -> Mux/3
  [T47_3739_3329394084968] -> Mux/4
  [T47_3740_3331932813404] -> Mux/5
  [T47_3741_3334597009500] -> Mux/6

== system IEEE123_4subsystem/powergui/EquivalentModel10/Sources ==
  Mux : Mux  Inputs=[1 1 1 1 1 1 1 1 1 1 1 1 1 1 1 1 1 1 1 1 1 1 1 1 1 1 1 1 1 1 1 1 1 1 1 1 1 1 1 1 1 1 1 1 1 1 1 1 1 1 1 1 1 1 1 1 1 1 1 1 1 1 1 1 1 1 1 1 1 1 3]
  Mux_u : Mux  Inputs=[6 73]
  SwitchCurrents : Constant  Value=zeros(6,1)
  u : Outport  VectorParamsAs1DForOutWhenUnconnected=off
  wires:
  Mux_u/1 -> u/1
  SwitchCurrents/1 -> Mux_u/1
  Mux/1 -> Mux_u/2
  [T171_14645_41209454772312] -> Mux/1
  [T172_14696_41436240274319] -> Mux/2
  [T141_12056_28544058289867] -> Mux/3
  [T141_12058_28573443141791] -> Mux/4
  [T141_12060_28603654685928] -> Mux/5
  [T141_12062_28634692922278] -> Mux/6
  [T171_14646_41206119581260] -> Mux/7
  [T172_14697_41432898649708] -> Mux/8
  [T141_12057_28542452630377] -> Mux/9
  [T141_12059_28571833882745] -> Mux/10
  [T141_12061_28602041827325] -> Mux/11
  [T141_12063_28633076464119] -> Mux/12
  [T171_14647_41202910164359] -> Mux/13
  [T172_14698_41429682068003] -> Mux/14
  [T141_12058_28540999505496] -> Mux/15
  [T141_12060_28570377158308] -> Mux/16
  [T141_12062_28600581503332] -> Mux/17
  [T141_12064_28631612540569] -> Mux/18
  [T148_12706_30522789445863] -> Mux/19
  [T149_12757_30768162839671] -> Mux/20
  [T118_10117_19796551939482] -> Mux/21
  [T118_10119_19819974132181] -> Mux/22
  [T118_10121_19844068524515] -> Mux/23
  [T118_10123_19868835116483] -> Mux/24
  [T74_6070_7885008289087] -> Mux/25
  [T74_6071_7888989683934] -> Mux/26
  [T74_6072_7893174706888] -> Mux/27
  [T74_6071_7882993610154] -> Mux/28
  [T74_6072_7886973301779] -> Mux/29
  [T74_6073_7891156621512] -> Mux/30
  [T74_6071_7882782667466] -> Mux/31
  [T74_6072_7886762776862] -> Mux/32
  [T74_6073_7890946514367] -> Mux/33
  [T74_6072_7880767203638] -> Mux/34
  [T74_6073_7884745609813] -> Mux/35
  [T74_6074_7888927644097] -> Mux/36
  [T127_10812_22624354716203] -> Mux/37
  [T127_10813_22632716578841] -> Mux/38
  [T127_10813_22623946099839] -> Mux/39
  [T127_10814_22632305910770] -> Mux/40
  [T127_10814_22623706832923] -> Mux/41
  [T127_10815_22632064592147] -> Mux/42
  [T104_8873_14888978272319] -> Mux/43
  [T104_8874_14895574954171] -> Mux/44
  [T84_7399_12383202046420] -> Mux/45
  [T84_7400_12380547807589] -> Mux/46
  [T84_7401_12378001408996] -> Mux/47
  [T84_7402_12375088265409] -> Mux/48
  [T84_7403_12372431935760] -> Mux/49
  [T84_7404_12369883446350] -> Mux/50
  [T159_13593_34857685669346] -> Mux/51
  [T160_13644_34974482730430] -> Mux/52
  [T159_13594_34855016103098] -> Mux/53
  [T160_13645_34971805408803] -> Mux/54
  [T159_13595_34852481803392] -> Mux/55
  [T160_13646_34969262508301] -> Mux/56
  [T136_11654_25020480075215] -> Mux/57
  [T137_11705_25162107096471] -> Mux/58
  [T62_5018_5096134607924] -> Mux/59
  [T62_5019_5099875124434] -> Mux/60
  [T62_5020_5103791332557] -> Mux/61
  [T62_5019_5094980155254] -> Mux/62
  [T62_5020_5098718603334] -> Mux/63
  [T62_5021_5102632743027] -> Mux/64
  [T62_5019_5094419525957] -> Mux/65
  [T62_5020_5098158481388] -> Mux/66
  [T62_5021_5102073128432] -> Mux/67
  [T62_5020_5093263952187] -> Mux/68
  [T62_5021_5097000839188] -> Mux/69
  [T62_5022_5100913417803] -> Mux/70
  [T44_3534_3292874153890] -> Mux/71

== system IEEE123_4subsystem/powergui/EquivalentModel10/State-Space ==
  In1 : Inport
  In2 : Inport  Port=2
  ssn_sfun_sw1 : S-Function  FunctionName=ssn_sfun_v1  Parameters=10,0  SFunctionDeploymentMode=off  EnableBusSupport=off  SFcnStateName=MOV_segment89,xn_g1,xn_g2,xn_g3,xn_g4,xn_g5,xn_g6,xn_g7,xn_g8,MOV_segment89,MOV_segment89,MOV_segment89,MOV_segment89,MOV_segment89,MOV_segment89,MOV_segment89,MOV_segment89,MOV_segment89,MOV_segment89,MOV_segment89,MOV_segment89,MOV_segment89,MOV_segment89,MOV_segment89,MOV_segment89,MOV_segment89,MOV_segment89,MOV_segment89,MOV_segment89,MOV_segment89,MOV_segment89,MOV_segment89,MOV_segment89,MOV_segment89,MOV_segment89,MOV_segment89,MOV_segment89,MOV_segment89,MOV_segment89,MOV_segment89,MOV_segment89,MOV_segment89,MOV_segment89,MOV_segment89,MOV_segment89,MOV_segment89,MOV_segment89,MOV_segment89,MOV_segment89,MOV_segment89,MOV_segment89,MOV_segment89,MOV_segment89,MOV_segment89,MOV_segment89,MOV_segment89,MOV_segment89,MOV_segment89,MOV_segment89,MOV_segment89,MOV_segment89,MOV_segment89,MOV_segment89,MOV_segment89,MOV_segment89,MOV_segment89,MOV_segment89,MOV_segment89,MOV_segment89,MOV_segment89,MOV_segment89,MOV_segment89,MOV_segment89,MOV_segment89,MOV_segment89,MOV_segment89,MOV_segment89,MOV_segment89,MOV_segment89,MOV_segment89,MOV_segment89,MOV_segment89,MOV_segment89,MOV_segment89,MOV_segment89,MOV_segment89,MOV_segment89,MOV_segment89,MOV_segment89,MOV_segment89
      settings: SFcnIsStateOwnerBlock=on
  Out1 : Outport  VectorParamsAs1DForOutWhenUnconnected=off
  Out2 : Outport  Port=2  VectorParamsAs1DForOutWhenUnconnected=off
  tag scope: ssn_ext_sys_from_V_201x9172x689cf8bd979c=global, ssn_ext_sys_from_V_89bxbdb6x1398f6ae2864=global, ssn_ext_sys_from_V_987xa5e3xeb9000d249b6=global, ssn_ext_sys_from_V_e52xa76ex313cf843a804=global
  wires:
  ssn_sfun_sw1/2 -> Out2/1
  In2/1 -> ssn_sfun_sw1/2
  ssn_sfun_sw1/1 -> Out1/1
  In1/1 -> ssn_sfun_sw1/1
  [ssn_ext_sys_goto_Hist_201x9172x689cf8bd979c] -> ssn_sfun_sw1/3
  [ssn_ext_sys_goto_Y_201x9172x689cf8bd979c] -> ssn_sfun_sw1/4
  ssn_sfun_sw1/3 -> [ssn_ext_sys_from_V_201x9172x689cf8bd979c]
  [ssn_ext_sys_goto_Hist_987xa5e3xeb9000d249b6] -> ssn_sfun_sw1/5
  [ssn_ext_sys_goto_Y_987xa5e3xeb9000d249b6] -> ssn_sfun_sw1/6
  ssn_sfun_sw1/4 -> [ssn_ext_sys_from_V_987xa5e3xeb9000d249b6]
  [ssn_ext_sys_goto_Hist_e52xa76ex313cf843a804] -> ssn_sfun_sw1/7
  [ssn_ext_sys_goto_Y_e52xa76ex313cf843a804] -> ssn_sfun_sw1/8
  ssn_sfun_sw1/5 -> [ssn_ext_sys_from_V_e52xa76ex313cf843a804]
  [ssn_ext_sys_goto_Hist_89bxbdb6x1398f6ae2864] -> ssn_sfun_sw1/9
  [ssn_ext_sys_goto_Y_89bxbdb6x1398f6ae2864] -> ssn_sfun_sw1/10
  ssn_sfun_sw1/6 -> [ssn_ext_sys_from_V_89bxbdb6x1398f6ae2864]

== system IEEE123_4subsystem/powergui/EquivalentModel10/Status ==
  status : Inport
  Demux : Demux  Outputs=[1 1 1 1 1 1]
  tag scope: T49_3974_4087805351122=global, T49_3975_4089788506250=global, T49_3976_4091892007908=global, T50_4027_4228564836506=global, T50_4028_4230675539592=global, T50_4029_4232909897078=global
  wires:
  status/1 -> Demux/1
  Demux/1 -> [T50_4027_4228564836506]
  Demux/2 -> [T50_4028_4230675539592]
  Demux/3 -> [T50_4029_4232909897078]
  Demux/4 -> [T49_3974_4087805351122]
  Demux/5 -> [T49_3975_4089788506250]
  Demux/6 -> [T49_3976_4091892007908]
